simulink library "dsplp"  (Simulink 6.0)
values from neighbouring files (symbols this model uses):
  range = max([ymax-ymin xmax-xmin])*excessRange    [sdspfscope2.m]
undefined symbols (not defined in the file or in its folder): D
libraries: dspsigattribs x3, dspsolvers x2, simulink x2, dspstat3 x1
settings Model: RequirementInfo=9  CovMetricSettings=d  Creator=szlotkin  LastModifiedBy=sconahan  ExtModeAutoUpdateStatusClock=off

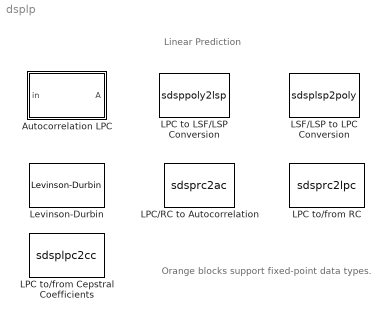
== system dsplp ==
  note: Linear Prediction
  note: Orange blocks support fixed-point data types.
  Autocorrelation LPC : Subsystem  mask(Autocorrelation LPC){lpcCoeffOutFcn=A, lpcOutP=off, inherit_prediction_order=off, order=1}
      mask prompts: lpcCoeffOutFcn "Output(s):"; lpcOutP "Output prediction error power (P)"; inherit_prediction_order "Inherit prediction order from input dimensions"; order "Prediction order (N):"
      mask help:
      | Output the coefficients of an Nth order forward linear predictor such that the sum of the squares of the errors is minimized (using the auto-
      | correlation LPC method).  The prediction coefficients are given in A (polynomial coefficients) and/or K (reflection coefficients).  The prediction error power is given in the optional P output.
      mask init:
      | acf = dspblklpc('init', order);
      mask Help: web(dspbhelp);
      mask StyleString: popup(A and K|A|K),checkbox,checkbox,edit
      mask CallbackString: ||acf = dspblklpc;|
      mask Display: disp('Autocorr\nLPC')
  LPC to LSF/LSP Conversion : S-Function  FunctionName=sdsppoly2lsp  Parameters=output,NSteps, NBisects, RootStatus,correction,lastLSP,lspvector,error  mask(LPC to LSF/LSP Conversion){output=LSP in range (-1 1), NSteps=64, NBisects=4, RootStatus=off, correction=off, lastLSP=off, lspvector=, error=Ignore}
      mask prompts: NSteps "Root finding coarse grid points:"; NBisects "Root finding bisection refinement:"; RootStatus "Show output validity status"; correction "If current output is invalid, overwrite with previous output"; lastLSP "When first output is invalid, overwrite with user-defined values"; lspvector "User-defined LSF/LSP values for overwriting invalid first output:"; error "If first input value is not 1:"
      mask help:
      | Convert linear prediction coefficients (LPCs) to line spectral pairs (LSPs) or line spectral frequencies (LSFs).  An optional output indicates the validity of the current output. Outputs can be invalid due to unstable inputs, or failure to find all LSF/LSPs.
      |
      | The first input coefficient must be 1.  If it is not, the block normalizes the input by default, and optionally gives a warning.
      mask init:
      | [si,so] = dspblkpoly2lsp('icon', RootStatus);
      | disp([ ])
      mask Help: web(dspbhelp);
      mask StyleString: popup(LSP in range (-1 1)|LSF normalized in range (0 0.5)|LSF in range (0 pi)),edit,edit,checkbox,checkbox,checkbox,edit,popup(Ignore|Normalize|Normalize and warn|Error)
      mask CallbackString: ||||dspblkpoly2lsp|dspblkpoly2lsp||
      mask Display:
      | port_label('input',si(1).port, si(1).txt);
      | port_label('output',so(1).port, so(1).txt);
      | port_label('output',so(2).port, so(2).txt);
  "LPC to/from Cepstral Coefficients " : S-Function  AncestorBlock=dsplp/LPC to//from RC  FunctionName=sdsplpc2cc  Parameters=conversion, enerpp,outpower, sizecb, nceps, error  mask(LPC to/from Cepstral Coefficients){conversion=LPCs to Cepstral coefficients, enerpp=assume P equals 1, outpower=off, sizecb=off, nceps=10, error=Replace it with 1}
      mask prompts: conversion "Type of conversion:"; enerpp "Specify P:"; outpower "Output P"; sizecb "Output size same as input size"; nceps "Length of output cepstral coefficient vector:"; error "If first input value is not 1:"
      mask help:
      | Converts linear prediction coefficients (LPCs) to/from cepstral coefficients (CCs).
      |
      | When converting from LPCs to CCs, you can assume the prediction error power is 1, or specify a different value using input port P. The size of the output vector of cepstral coefficients can be the same length as the input LPC vector, or you can define a nonzero length. The first input coefficient must be 1. If it is not, you can replace it with 1, normalize the input with the non-unity first coefficient, normalize and warn, or error out.
      |
      | When converting from CCs to LPCs, you can output the prediction error power at port P.
      mask init:
      | [si,so,icontxt] = dspblklpc2cc('icon');
      mask Help: web(dspbhelp);
      mask StyleString: popup(LPCs to cepstral coefficients|Cepstral coefficients to LPCs),popup(assume P equals 1|via input port),checkbox,checkbox,edit,popup(Replace it with 1|Normalize|Normalize and warn|Error)
      mask CallbackString: dspblklpc2cc|||dspblklpc2cc||
      mask Display:
      | disp(icontxt)
      | port_label('input',si(1).port, si(1).txt);
      | port_label('input',si(2).port, si(2).txt);
      | port_label('output',so(1).port, so(1).txt);
      | port_label('output',so(2).port, so(2).txt);
  LPC to/from RC : S-Function  FunctionName=sdsprc2lpc  Parameters=conversion, perr, stability, error  mask(LPC to/from RC){conversion=RC to LPC, perr=on, stability=off, error=Replace it with 1}
      mask prompts: conversion "Type of conversion"; perr "Output normalized prediction error power"; stability "Output LPC filter stability"; error "If first input value is not 1:"
      mask help:
      | Converts Linear Prediction polynomial coefficients (A) to/from Reflection coefficients (K). The normalized prediction error power of the linear prediciton filter is given in the optional P output. The stability of the prediction coefficients is given in the optional S output.
      | In the LPC to RC conversion, the first input coefficient must be 1. If it is not, you can optionally replace it with 1, or normalize the input with the non-unity 1st coefficient and warn, or error out.
      mask init:
      | [si,so,icontxt] = dspblkrc2lpc('icon', perr, stability);
      mask Help: web(dspbhelp);
      mask StyleString: popup(RC to LPC|LPC to RC),checkbox,checkbox,popup(Replace it with 1|Normalize|Normalize and warn|Error)
      mask CallbackString: dspblkrc2lpc|||
      mask Display:
      | disp(icontxt)
      | port_label('input',si(1).port, si(1).txt);
      | port_label('output',so(1).port, so(1).txt);
      | port_label('output',so(2).port, so(2).txt);
      | port_label('output',so(3).port, so(3).txt);
  LPC/RC to Autocorrelation : S-Function  FunctionName=sdsprc2ac  Parameters=conversion, perr_spec, error  mask(LPC/RC to Autocorrelation){conversion=LPC to autocorrelation, perr_spec=Assume P = 1, error=Replace it with 1}
      mask prompts: conversion "Type of conversion"; perr_spec "Specify P:"; error "If first input value is not 1:"
      mask help:
      | Converts Linear Prediction Coefficients (A) or Reflection Coefficients (K) into Autocorrelation coefficients (AC). We can have an optional prediction error power (P) input port which expects a scalar value, in the absence of which P is assumed to be 1.
      |
      | In the LPC to Autocorrelation coefficient conversion, the first input coefficient is expected to be 1. If it is not, user can select one of 4 options, like replace the first coefficient with 1, or normalize the input vector with first coefficient, or normalize and warn, or just error out.
      mask init:
      | [si,so, icontxt] = dspblkrc2ac('icon',perr_spec);
      | disp([ ])
      mask Help: web(dspbhelp);
      mask StyleString: popup(LPC to autocorrelation|RC to autocorrelation),popup(Assume P = 1|Via input port),popup(Replace it with 1|Normalize|Normalize and warn|Error)
      mask CallbackString: dspblkrc2ac||
      mask Display:
      | disp(icontxt)
      | port_label('input',si(1).port, si(1).txt);
      | port_label('input',si(2).port, si(2).txt);
      | port_label('output',so(1).port, so(1).txt);
  LSF/LSP to LPC Conversion : S-Function  FunctionName=sdsplsp2poly  Parameters=input  mask(LSF/LSP to LPC Conversion){input=LSP in range (-1 1)}
      mask help: Convert line spectral frequencies (LSFs) or line spectral pairs (LSPs) to linear prediction coefficients (LPCs). The LSF inputs can be in the range (0 pi), or normalized to be in the range (0 0.5).
      mask init:
      | [si,so] = dspblklsp2poly('icon');
      mask Help: web(dspbhelp);
      mask StyleString: popup(LSP in range (-1 1)|LSF normalized in range (0 0.5)|LSF in range (0 pi))
      mask Display:
      | port_label('input',si(1).port, si(1).txt);
      | port_label('output',so(1).port, so(1).txt);
  Levinson-Durbin : dspsolvers/Levinson-Durbin  coeffOutFcn=K  outP=off  zeroInpHandling=on  firstCoeffMode=Binary point scaling  firstCoeffWordLength=16  firstCoeffFracLength=15  secondCoeffMode=Binary point scaling  secondCoeffWordLength=16  secondCoeffFracLength=15  accumMode=User-defined  accumWordLength=32  accumFracLength=30  prodOutputMode=User-defined  prodOutputWordLength=32  prodOutputFracLength=30  roundingMode=Floor  overflowMode=off
      settings: allowOverrides=off

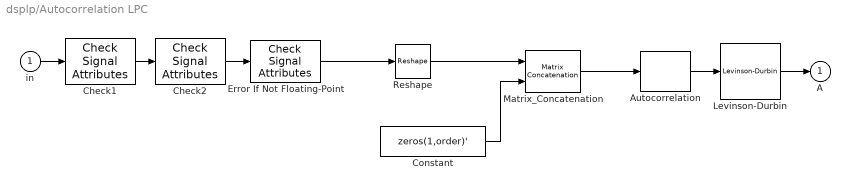
== system dsplp/Autocorrelation LPC ==
  in : Inport
  Autocorrelation : dspstat3/Autocorrelation  DialogController=dspDDGCreate  DialogControllerArgs=DataTag0  AllPositiveLags=off  maxlag=acf  bias=Biased  domain=Time  roundingMode=Floor  overflowMode=off
  "Check1 " : dspsigattribs/Check Signal Attributes  SigAttribCheckMethod=Does not match attributes exactly  Complexity=Ignore  Frame=Ignore  DimsCheckMethod=Is...  Dimensions=Vector (1-D or 2-D) or scalar  DatatypeCheckMethod=Ignore  DatatypeGeneral=Boolean  DtypeFloatSpecific=Any floating-point  DtypeFixedSpecific=Any fixed-point  DtypeIntSpecific=Any integer  SampleMode=Ignore
  Check2 : dspsigattribs/Check Signal Attributes  SigAttribCheckMethod=Matches attributes exactly  Complexity=Ignore  Frame=Frame-based  DimsCheckMethod=Is...  Dimensions=Row vector (2-D)  DatatypeCheckMethod=Ignore  DatatypeGeneral=Boolean  DtypeFloatSpecific=Any floating-point  DtypeFixedSpecific=Any fixed-point  DtypeIntSpecific=Any integer  SampleMode=Ignore
  Constant : Constant  Value=zeros(1,order)'
  Error If Not Floating-Point : dspsigattribs/Check Signal Attributes  SigAttribCheckMethod=Does not match attributes exactly  Complexity=Ignore  Frame=Ignore  DimsCheckMethod=Ignore  Dimensions=1-D  DatatypeCheckMethod=Is...  DatatypeGeneral=Floating-point  DtypeFloatSpecific=Any floating-point  DtypeFixedSpecific=Any fixed-point  DtypeIntSpecific=Any integer  SampleMode=Ignore
  Levinson-Durbin : dspsolvers/Levinson-Durbin  coeffOutFcn=A  outP=off  zeroInpHandling=on  firstCoeffMode=Binary point scaling  firstCoeffWordLength=16  firstCoeffFracLength=15  secondCoeffMode=Binary point scaling  secondCoeffWordLength=16  secondCoeffFracLength=15  accumMode=User-defined  accumWordLength=32  accumFracLength=30  prodOutputMode=User-defined  prodOutputWordLength=32  prodOutputFracLength=30  roundingMode=Floor  overflowMode=off
      settings: allowOverrides=off
  Matrix_Concatenation : simulink/Math Operations/Matrix Concatenation  numInports=2  catMethod=Vertical
  Reshape : simulink/Math Operations/Reshape  OutputDimensionality=Column vector  OutputDimensions=[1,1]
  A : Outport  InitialOutput=0
  wires:
  Reshape/1 -> Matrix_Concatenation/1
  in/1 -> "Check1 "/1
  Autocorrelation/1 -> Levinson-Durbin/1
  Levinson-Durbin/1 -> A/1
  "Check1 "/1 -> Check2/1
  Check2/1 -> Error If Not Floating-Point/1
  Matrix_Concatenation/1 -> Autocorrelation/1
  Constant/1 -> Matrix_Concatenation/2
  Error If Not Floating-Point/1 -> Reshape/1
